simulink model "EKF"  (R2018b)
settings: Solver=ode45  StartTime=0.0  StopTime=900  MaxStep=0.001  RelTol=1e-3
libraries: simulink x9
settings Model: Creator=LaAir  LastModifiedBy=LaAir

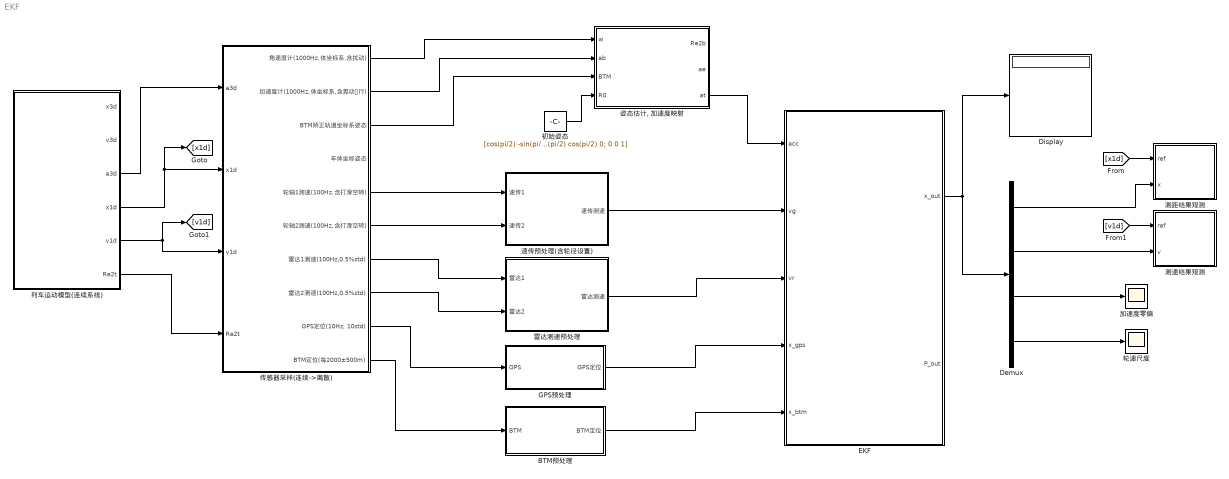
== system EKF ==
  BTM预处理 : Subsystem
  Demux : Demux
  Display : Display
  EKF : MATLAB Function  TreatAsAtomicUnit=on  SystemSampleTime=1e-3
  GPS预处理 : Subsystem
  传感器采样(连续->离散) : Subsystem
  列车运动模型(连续系统) : Subsystem
  初始姿态 : Constant  Value=[cos(pi/2) -sin(pi/2) 0; sin(pi/2) cos(pi/2) 0; 0 0 1]
  加速度零偏 : Scope
  "姿态估计, 加速度映射" : Subsystem
  测距结果观测 : Subsystem
  测速结果观测 : Subsystem
  轮速尺度 : Scope
  速传预处理(含轮径设置) : Subsystem
  雷达测速预处理 : Subsystem
  wires:
  速传预处理(含轮径设置)/1(速传测速) -> EKF/2(vg)
  雷达测速预处理/1(雷达测速) -> EKF/3(vr)
  BTM预处理/1(BTM定位) -> EKF/5(x_btm)
  GPS预处理/1(GPS定位) -> EKF/4(x_gps)
  列车运动模型(连续系统)/5(v1d) -> [v1d], 传感器采样(连续->离散)/3(v1d)
  列车运动模型(连续系统)/4(x1d) -> 传感器采样(连续->离散)/2(x1d), [x1d]
  列车运动模型(连续系统)/3(a3d) -> 传感器采样(连续->离散)/1(a3d)
  传感器采样(连续->离散)/5(轮轴1测速(100Hz,含打滑空转)) -> 速传预处理(含轮径设置)/1(速传1)
  传感器采样(连续->离散)/10(BTM定位(每2000±500m)) -> BTM预处理/1(BTM)
  列车运动模型(连续系统)/6(Re2t) -> 传感器采样(连续->离散)/4(Re2t)
  传感器采样(连续->离散)/9("GPS定位(10Hz, 10std)") -> GPS预处理/1(GPS)
  传感器采样(连续->离散)/7(雷达1测速(100Hz,0.5%std)) -> 雷达测速预处理/1(雷达1)
  传感器采样(连续->离散)/6(轮轴2测速(100Hz,含打滑空转)) -> 速传预处理(含轮径设置)/2(速传2)
  传感器采样(连续->离散)/8(雷达2测速(100Hz,0.5%std)) -> 雷达测速预处理/2(雷达2)
  初始姿态/1 -> "姿态估计, 加速度映射"/4(R0)
  传感器采样(连续->离散)/1(角速度计(1000Hz,体坐标系,含扰动)) -> "姿态估计, 加速度映射"/1(w)
  传感器采样(连续->离散)/2(加速度计(1000Hz,体坐标系,含晃动🐍行)) -> "姿态估计, 加速度映射"/2(ab)
  传感器采样(连续->离散)/3(BTM矫正轨道坐标系姿态) -> "姿态估计, 加速度映射"/3(BTM)
  EKF/1(x_out) -> Demux/1, Display/1
  [x1d] -> 测距结果观测/1(ref)
  [v1d] -> 测速结果观测/1(ref)
  Demux/1 -> 测距结果观测/2(x)
  Demux/2 -> 测速结果观测/2(v)
  Demux/3 -> 加速度零偏/1
  Demux/4 -> 轮速尺度/1
  "姿态估计, 加速度映射"/3(at) -> EKF/1(acc)

== system EKF/BTM预处理 ==
  note: 需将最后输出的采样频率与主融合器保持一致(1000Hz)
  BTM : Inport
  1000Hz : ZeroOrderHold  SampleTime=1e-3
  Pulse Holder (1000Hz) : Subsystem
  BTM定位 : Outport
  wires:
  BTM/1 -> 1000Hz/1
  1000Hz/1 -> Pulse Holder (1000Hz)/1(I)
  Pulse Holder (1000Hz)/1(O) -> BTM定位/1

== system EKF/GPS预处理 ==
  note: 需将最后输出的采样频率与主融合器保持一致(1000Hz)
  GPS : Inport
  Pulse Holder (1000Hz) : Subsystem
  GPS定位 : Outport
  wires:
  GPS/1 -> Pulse Holder (1000Hz)/1(I)
  Pulse Holder (1000Hz)/1(O) -> GPS定位/1

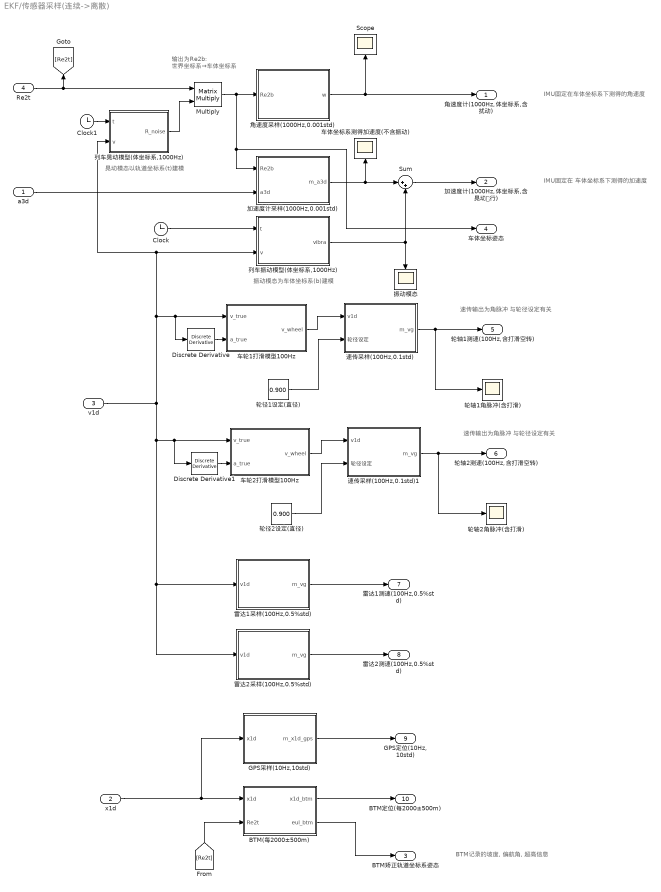
== system EKF/传感器采样(连续->离散) ==
  note: 速传输出为角脉冲
      | 与轮径设定有关
  note: 速传输出为角脉冲
      | 与轮径设定有关
  note: 输出为Re2b:
      | 世界坐标系→车体坐标系
  note: IMU固定在车体坐标系下测得的角速度
  note: IMU固定在 车体坐标系下测得的加速度
  note: 振动模态为车体坐标系(b)建模
  note: 晃动模态以轨道坐标系(t)建模
  note: BTM记录的坡度, 偏航角, 超高信息
  a3d : Inport
  x1d : Inport  Port=2
  v1d : Inport  Port=3
  Re2t : Inport  Port=4
  BTM(每2000±500m) : Subsystem
  Clock : Clock
  Clock1 : Clock
  Discrete Derivative : simulink/Discrete/Discrete Derivative  gainval=1.0  ICPrevScaledInput=0.0  OutMin=[]  OutMax=[]  OutDataType=fixdt(1, 16)  OutScaling=2^-10  DoSatur=off
  Discrete Derivative1 : simulink/Discrete/Discrete Derivative  gainval=1.0  ICPrevScaledInput=0.0  OutMin=[]  OutMax=[]  OutDataType=fixdt(1, 16)  OutScaling=2^-10  DoSatur=off
  GPS采样(10Hz,10std) : Subsystem
  Multiply : Product  Multiplication=Matrix(*)
  Scope : Scope
  Sum : Sum  Inputs=|++
  列车振动模型(体坐标系,1000Hz) : MATLAB Function  TreatAsAtomicUnit=on  SystemSampleTime=1e-3
  列车晃动模型(体坐标系,1000Hz) : MATLAB Function  TreatAsAtomicUnit=on  SystemSampleTime=1e-3
  加速度计采样(1000Hz,0.001std) : Subsystem
  振动模态 : Scope
  角速度采样(1000Hz,0.001std) : Subsystem
  车体坐标系测得加速度(不含振动) : Scope
  车轮1打滑模型100Hz : MATLAB Function  TreatAsAtomicUnit=on  SystemSampleTime=1e-2
  车轮2打滑模型100Hz : MATLAB Function  TreatAsAtomicUnit=on  SystemSampleTime=1e-2
  轮径1设定(直径) : Constant  Value=0.900
  轮径2设定(直径) : Constant  Value=0.900
  轮轴1角脉冲(含打滑) : Scope
  轮轴2角脉冲(含打滑) : Scope
  速传采样(100Hz,0.1std) : Subsystem
  速传采样(100Hz,0.1std)1 : Subsystem
  雷达1采样(100Hz,0.5%std) : Subsystem
  雷达2采样(100Hz,0.5%std) : Subsystem
  角速度计(1000Hz,体坐标系,含扰动) : Outport
  加速度计(1000Hz,体坐标系,含晃动🐍行) : Outport  Port=2
  BTM矫正轨道坐标系姿态 : Outport  Port=3
  车体坐标姿态 : Outport  Port=4
  轮轴1测速(100Hz,含打滑空转) : Outport  Port=5
  轮轴2测速(100Hz,含打滑空转) : Outport  Port=6
  雷达1测速(100Hz,0.5%std) : Outport  Port=7
  雷达2测速(100Hz,0.5%std) : Outport  Port=8
  "GPS定位(10Hz, 10std)" : Outport  Port=9
  BTM定位(每2000±500m) : Outport  Port=10
  wires:
  x1d/1 -> GPS采样(10Hz,10std)/1(x1d), BTM(每2000±500m)/1(x1d)
  BTM(每2000±500m)/1(x1d_btm) -> BTM定位(每2000±500m)/1
  速传采样(100Hz,0.1std)/1(m_vg) -> 轮轴1角脉冲(含打滑)/1, 轮轴1测速(100Hz,含打滑空转)/1
  GPS采样(10Hz,10std)/1(m_x1d_gps) -> "GPS定位(10Hz, 10std)"/1
  a3d/1 -> 加速度计采样(1000Hz,0.001std)/2(a3d)
  轮径1设定(直径)/1 -> 速传采样(100Hz,0.1std)/2(轮径设定)
  雷达1采样(100Hz,0.5%std)/1(m_vg) -> 雷达1测速(100Hz,0.5%std)/1
  Discrete Derivative/1 -> 车轮1打滑模型100Hz/2(a_true)
  车轮1打滑模型100Hz/1(v_wheel) -> 速传采样(100Hz,0.1std)/1(v1d)
  Clock/1 -> 列车振动模型(体坐标系,1000Hz)/1(t)
  加速度计采样(1000Hz,0.001std)/1(m_a3d) -> 车体坐标系测得加速度(不含振动)/1, Sum/1
  Sum/1 -> 加速度计(1000Hz,体坐标系,含晃动🐍行)/1
  列车振动模型(体坐标系,1000Hz)/1(vibra) -> Sum/2, 振动模态/1
  车轮2打滑模型100Hz/1(v_wheel) -> 速传采样(100Hz,0.1std)1/1(v1d)
  轮径2设定(直径)/1 -> 速传采样(100Hz,0.1std)1/2(轮径设定)
  Discrete Derivative1/1 -> 车轮2打滑模型100Hz/2(a_true)
  速传采样(100Hz,0.1std)1/1(m_vg) -> 轮轴2角脉冲(含打滑)/1, 轮轴2测速(100Hz,含打滑空转)/1
  v1d/1 -> Discrete Derivative1/1, 车轮2打滑模型100Hz/1(v_true), 雷达2采样(100Hz,0.5%std)/1(v1d), 雷达1采样(100Hz,0.5%std)/1(v1d), 列车晃动模型(体坐标系,1000Hz)/2(v), 列车振动模型(体坐标系,1000Hz)/2(v), Discrete Derivative/1, 车轮1打滑模型100Hz/1(v_true)
  雷达2采样(100Hz,0.5%std)/1(m_vg) -> 雷达2测速(100Hz,0.5%std)/1
  Re2t/1 -> Multiply/1, [Re2t]
  列车晃动模型(体坐标系,1000Hz)/1(R_noise) -> Multiply/2
  Clock1/1 -> 列车晃动模型(体坐标系,1000Hz)/1(t)
  Multiply/1 -> 角速度采样(1000Hz,0.001std)/1(Re2b), 车体坐标姿态/1, 加速度计采样(1000Hz,0.001std)/1(Re2b)
  角速度采样(1000Hz,0.001std)/1(w) -> 角速度计(1000Hz,体坐标系,含扰动)/1, Scope/1
  BTM(每2000±500m)/2(eul_btm) -> BTM矫正轨道坐标系姿态/1
  [Re2t] -> BTM(每2000±500m)/2(Re2t)

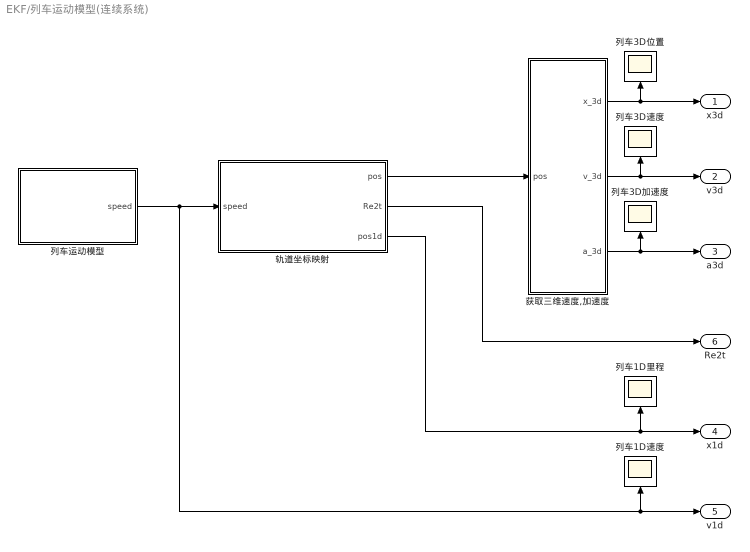
== system EKF/列车运动模型(连续系统) ==
  列车1D速度 : Scope
  列车1D里程 : Scope
  列车3D位置 : Scope
  列车3D加速度 : Scope
  列车3D速度 : Scope
  列车运动模型 : Subsystem
  获取三维速度,加速度 : Subsystem
  轨道坐标映射 : Subsystem
  x3d : Outport
  v3d : Outport  Port=2
  a3d : Outport  Port=3
  x1d : Outport  Port=4
  v1d : Outport  Port=5
  Re2t : Outport  Port=6
  wires:
  轨道坐标映射/1(pos) -> 获取三维速度,加速度/1(pos)
  获取三维速度,加速度/1(x_3d) -> 列车3D位置/1, x3d/1
  列车运动模型/1(speed) -> 轨道坐标映射/1(speed), 列车1D速度/1, v1d/1
  获取三维速度,加速度/3(a_3d) -> 列车3D加速度/1, a3d/1
  获取三维速度,加速度/2(v_3d) -> 列车3D速度/1, v3d/1
  轨道坐标映射/3(pos1d) -> x1d/1, 列车1D里程/1
  轨道坐标映射/2(Re2t) -> Re2t/1

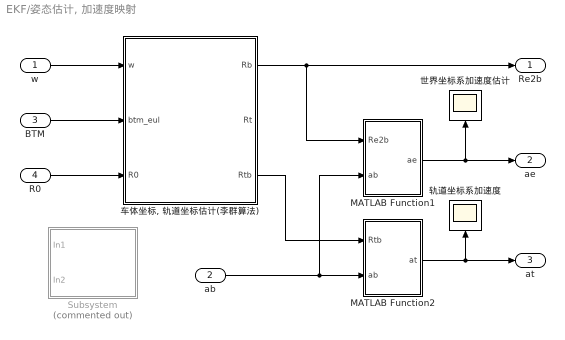
== system EKF/姿态估计, 加速度映射 ==
  w : Inport
  ab : Inport  Port=2
  BTM : Inport  Port=3
  R0 : Inport  Port=4
  MATLAB Function1 : MATLAB Function  TreatAsAtomicUnit=on
  MATLAB Function2 : MATLAB Function  TreatAsAtomicUnit=on
  Subsystem : Subsystem  Commented=on
  世界坐标系加速度估计 : Scope
  "车体坐标, 轨道坐标估计(李群算法)" : MATLAB Function  TreatAsAtomicUnit=on  SystemSampleTime=1e-3
  轨道坐标系加速度 : Scope
  Re2b : Outport
  ae : Outport  Port=2
  at : Outport  Port=3
  wires:
  "车体坐标, 轨道坐标估计(李群算法)"/1(Rb) -> Re2b/1, MATLAB Function1/1(Re2b)
  ab/1 -> MATLAB Function2/2(ab), MATLAB Function1/2(ab)
  R0/1 -> "车体坐标, 轨道坐标估计(李群算法)"/3(R0)
  w/1 -> "车体坐标, 轨道坐标估计(李群算法)"/1(w)
  BTM/1 -> "车体坐标, 轨道坐标估计(李群算法)"/2(btm_eul)
  MATLAB Function1/1(ae) -> ae/1, 世界坐标系加速度估计/1
  "车体坐标, 轨道坐标估计(李群算法)"/3(Rtb) -> MATLAB Function2/1(Rtb)
  MATLAB Function2/1(at) -> at/1, 轨道坐标系加速度/1

== system EKF/测距结果观测 ==
  ref : Inport
  x : Inport  Port=2
  BTM开窗失败 : MATLAB Function  TreatAsAtomicUnit=on
  EKF测距偏差 : Scope
  EKF测距对比 : Scope  NumInputPorts=2
  Scope : Scope
  Sum : Sum  Inputs=+-
  wires:
  x/1 -> EKF测距对比/2, Sum/2
  Sum/1 -> BTM开窗失败/1(u), EKF测距偏差/1
  ref/1 -> Sum/1, EKF测距对比/1
  BTM开窗失败/1(y) -> Scope/1

== system EKF/测速结果观测 ==
  ref : Inport
  v : Inport  Port=2
  EKF测速偏差 : Scope
  EKF速度对比 : Scope  NumInputPorts=2
  Sum : Sum  Inputs=+-
  wires:
  v/1 -> EKF速度对比/2, Sum/2
  Sum/1 -> EKF测速偏差/1
  ref/1 -> Sum/1, EKF速度对比/1

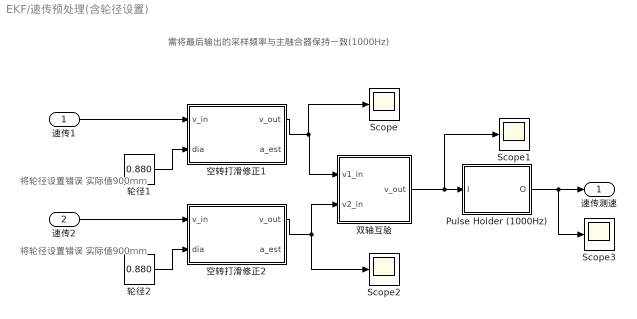
== system EKF/速传预处理(含轮径设置) ==
  note: 将轮径设置错误
      | 实际值900mm
  note: 将轮径设置错误
      | 实际值900mm
  note: 需将最后输出的采样频率与主融合器保持一致(1000Hz)
  速传1 : Inport
  速传2 : Inport  Port=2
  Pulse Holder (1000Hz) : Subsystem
  Scope{,1..3} (4 alike) : Scope
  双轴互验 : MATLAB Function  TreatAsAtomicUnit=on  SystemSampleTime=1e-2
  空转打滑修正1 : MATLAB Function  TreatAsAtomicUnit=on  SystemSampleTime=1e-2
  空转打滑修正2 : MATLAB Function  TreatAsAtomicUnit=on  SystemSampleTime=1e-2
  轮径1 : Constant  Value=0.880
  轮径2 : Constant  Value=0.880
  速传测速 : Outport
  wires:
  轮径1/1 -> 空转打滑修正1/2(dia)
  空转打滑修正2/1(v_out) -> Scope2/1, 双轴互验/2(v2_in)
  双轴互验/1(v_out) -> Scope1/1, Pulse Holder (1000Hz)/1(I)
  空转打滑修正1/1(v_out) -> Scope/1, 双轴互验/1(v1_in)
  轮径2/1 -> 空转打滑修正2/2(dia)
  速传1/1 -> 空转打滑修正1/1(v_in)
  速传2/1 -> 空转打滑修正2/1(v_in)
  Pulse Holder (1000Hz)/1(O) -> Scope3/1, 速传测速/1

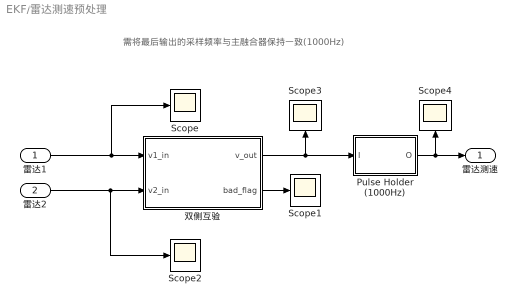
== system EKF/雷达测速预处理 ==
  note: 需将最后输出的采样频率与主融合器保持一致(1000Hz)
  雷达1 : Inport
  雷达2 : Inport  Port=2
  Pulse Holder (1000Hz) : Subsystem
  Scope{,1..4} (5 alike) : Scope
  双侧互验 : MATLAB Function  TreatAsAtomicUnit=on  SystemSampleTime=1e-2
  雷达测速 : Outport
  wires:
  雷达1/1 -> 双侧互验/1(v1_in), Scope/1
  雷达2/1 -> Scope2/1, 双侧互验/2(v2_in)
  双侧互验/1(v_out) -> Scope3/1, Pulse Holder (1000Hz)/1(I)
  双侧互验/2(bad_flag) -> Scope1/1
  Pulse Holder (1000Hz)/1(O) -> 雷达测速/1, Scope4/1

== system EKF/BTM预处理/Pulse Holder (1000Hz) ==
  I : Inport
  Multiply : Product
  pulse holder : Subsystem
  O : Outport
  wires:
  Multiply/1 -> O/1
  pulse holder/1(O) -> Multiply/2
  I/1 -> Multiply/1, pulse holder/1(I)

== system EKF/GPS预处理/Pulse Holder (1000Hz) ==
  I : Inport
  Multiply : Product
  pulse holder : Subsystem
  O : Outport
  wires:
  Multiply/1 -> O/1
  pulse holder/1(O) -> Multiply/2
  I/1 -> Multiply/1, pulse holder/1(I)

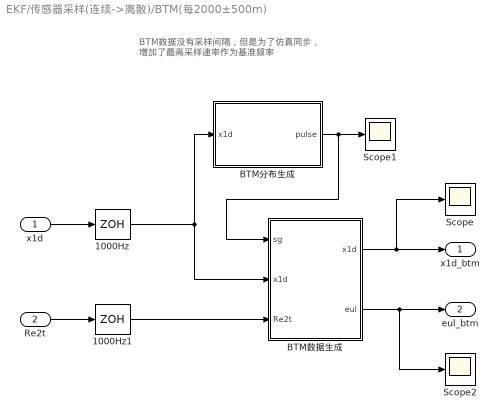
== system EKF/传感器采样(连续->离散)/BTM(每2000±500m) ==
  note: BTM数据没有采样间隔，但是为了仿真同步，
      | 增加了最高采样速率作为基准频率
  x1d : Inport
  Re2t : Inport  Port=2
  1000Hz : ZeroOrderHold  SampleTime=1e-3
  1000Hz1 : ZeroOrderHold  SampleTime=1e-3
  BTM分布生成 : MATLAB Function  TreatAsAtomicUnit=on  SystemSampleTime=1e-3
  BTM数据生成 : MATLAB Function  TreatAsAtomicUnit=on  SystemSampleTime=1e-3
  Scope : Scope
  Scope1 : Scope
  Scope2 : Scope
  x1d_btm : Outport
  eul_btm : Outport  Port=2
  wires:
  x1d/1 -> 1000Hz/1
  1000Hz/1 -> BTM数据生成/2("x1d "), BTM分布生成/1(x1d)
  Re2t/1 -> 1000Hz1/1
  BTM分布生成/1(pulse) -> BTM数据生成/1(sg), Scope1/1
  1000Hz1/1 -> BTM数据生成/3(Re2t)
  BTM数据生成/1(x1d) -> Scope/1, x1d_btm/1
  BTM数据生成/2(eul) -> Scope2/1, eul_btm/1

== system EKF/传感器采样(连续->离散)/GPS采样(10Hz,10std) ==
  x1d : Inport
  "10Hz, 10std" : simulink/Sources/Band-Limited White Noise  Cov=10  Ts=1e-1  seed=1006
  10hz采样 : ZeroOrderHold  SampleTime=1e-1
  GPS定位(10Hz,10std) : Scope
  Sum : Sum
  m_x1d_gps : Outport
  wires:
  x1d/1 -> 10hz采样/1
  "10Hz, 10std"/1 -> Sum/1
  10hz采样/1 -> Sum/2
  Sum/1 -> GPS定位(10Hz,10std)/1, m_x1d_gps/1

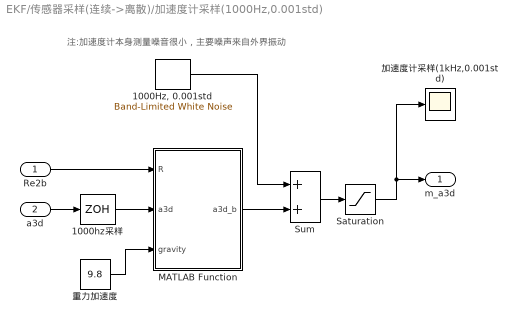
== system EKF/传感器采样(连续->离散)/加速度计采样(1000Hz,0.001std) ==
  note: 注:加速度计本身测量噪音很小，主要噪声来自外界振动
  Re2b : Inport
  a3d : Inport  Port=2
  "1000Hz, 0.001std" : simulink/Sources/Band-Limited White Noise  Cov=1e-9  Ts=1e-3  seed=1001
  1000hz采样 : ZeroOrderHold  SampleTime=1e-3
  MATLAB Function : MATLAB Function  TreatAsAtomicUnit=on
  Saturation : Saturate  UpperLimit=100  LowerLimit=-100
  Sum : Sum
  加速度计采样(1kHz,0.001std) : Scope
  重力加速度 : Constant  Value=9.8
  m_a3d : Outport
  wires:
  "1000Hz, 0.001std"/1 -> Sum/1
  MATLAB Function/1(a3d_b) -> Sum/2
  Sum/1 -> Saturation/1
  Re2b/1 -> MATLAB Function/1(R)
  a3d/1 -> 1000hz采样/1
  1000hz采样/1 -> MATLAB Function/2(a3d)
  重力加速度/1 -> MATLAB Function/3(gravity)
  Saturation/1 -> m_a3d/1, 加速度计采样(1kHz,0.001std)/1

== system EKF/传感器采样(连续->离散)/角速度采样(1000Hz,0.001std) ==
  Re2b : Inport
  "1000Hz, 1e-3std" : simulink/Sources/Band-Limited White Noise  Cov=1e-9  Ts=1e-3  seed=1010
  Sum1 : Sum
  角速度采样(1000Hz) : MATLAB Function  TreatAsAtomicUnit=on  SystemSampleTime=1e-3
  w : Outport
  wires:
  "1000Hz, 1e-3std"/1 -> Sum1/1
  角速度采样(1000Hz)/1(w) -> Sum1/2
  Sum1/1 -> w/1
  Re2b/1 -> 角速度采样(1000Hz)/1(R)

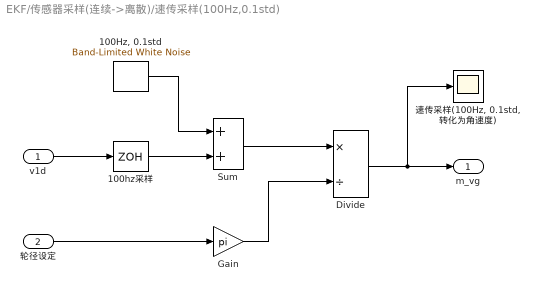
== system EKF/传感器采样(连续->离散)/速传采样(100Hz,0.1std) ==
  v1d : Inport
  轮径设定 : Inport  Port=2
  "100Hz, 0.1std" : simulink/Sources/Band-Limited White Noise  Cov=1e-4  Ts=1e-2  seed=1002
  100hz采样 : ZeroOrderHold  SampleTime=1e-2
  Divide : Product  Inputs=*/
  Gain : Gain  Gain=pi
  Sum : Sum
  "速传采样(100Hz, 0.1std, 转化为角速度)" : Scope
  m_vg : Outport
  wires:
  v1d/1 -> 100hz采样/1
  100hz采样/1 -> Sum/2
  Sum/1 -> Divide/1
  "100Hz, 0.1std"/1 -> Sum/1
  Divide/1 -> "速传采样(100Hz, 0.1std, 转化为角速度)"/1, m_vg/1
  Gain/1 -> Divide/2
  轮径设定/1 -> Gain/1

== system EKF/传感器采样(连续->离散)/速传采样(100Hz,0.1std)1 ==
  v1d : Inport
  轮径设定 : Inport  Port=2
  "100Hz, 0.1std" : simulink/Sources/Band-Limited White Noise  Cov=1e-4  Ts=1e-2  seed=1003
  100hz采样 : ZeroOrderHold  SampleTime=1e-2
  Divide : Product  Inputs=*/
  Gain : Gain  Gain=pi
  Sum : Sum
  "速传采样(100Hz, 0.1std, 转化为角速度)" : Scope
  m_vg : Outport
  wires:
  v1d/1 -> 100hz采样/1
  100hz采样/1 -> Sum/2
  Sum/1 -> Divide/1
  "100Hz, 0.1std"/1 -> Sum/1
  Divide/1 -> "速传采样(100Hz, 0.1std, 转化为角速度)"/1, m_vg/1
  Gain/1 -> Divide/2
  轮径设定/1 -> Gain/1

== system EKF/传感器采样(连续->离散)/雷达1采样(100Hz,0.5%std) ==
  v1d : Inport
  "100Hz, 0.005std" : simulink/Sources/Band-Limited White Noise  Cov=25e-8  Ts=1e-2  seed=1004
  100hz采样 : ZeroOrderHold  SampleTime=1e-2
  Multiply : Product
  Sum : Sum
  "速传采样(100Hz, 0.5%std)" : Scope
  m_vg : Outport
  wires:
  v1d/1 -> 100hz采样/1
  100hz采样/1 -> Multiply/2, Sum/2
  Sum/1 -> "速传采样(100Hz, 0.5%std)"/1, m_vg/1
  "100Hz, 0.005std"/1 -> Multiply/1
  Multiply/1 -> Sum/1

== system EKF/传感器采样(连续->离散)/雷达2采样(100Hz,0.5%std) ==
  v1d : Inport
  "100Hz, 0.005std" : simulink/Sources/Band-Limited White Noise  Cov=25e-8  Ts=1e-2  seed=1005
  100hz采样 : ZeroOrderHold  SampleTime=1e-2
  Multiply : Product
  Sum : Sum
  "速传采样(100Hz, 0.5%std)" : Scope
  m_vg : Outport
  wires:
  v1d/1 -> 100hz采样/1
  100hz采样/1 -> Multiply/2, Sum/2
  Sum/1 -> "速传采样(100Hz, 0.5%std)"/1, m_vg/1
  "100Hz, 0.005std"/1 -> Multiply/1
  Multiply/1 -> Sum/1

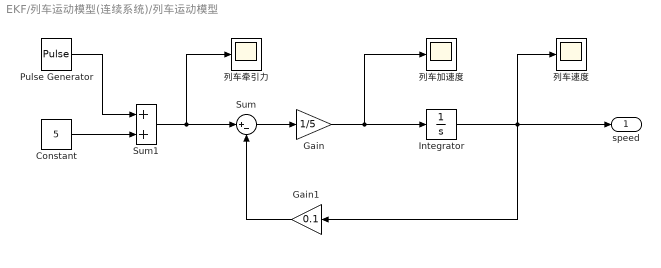
== system EKF/列车运动模型(连续系统)/列车运动模型 ==
  Constant : Constant  Value=5
  Gain : Gain  Gain=1/5
  Gain1 : Gain  Gain=0.1
  Integrator : Integrator
  Pulse Generator : DiscretePulseGenerator  PulseType=Time based  Amplitude=5  Period=600  PulseWidth=50
  Sum : Sum  Inputs=|+-
  Sum1 : Sum
  列车加速度 : Scope
  列车牵引力 : Scope
  列车速度 : Scope
  speed : Outport
  wires:
  Gain1/1 -> Sum/2
  Integrator/1 -> 列车速度/1, speed/1, Gain1/1
  Sum/1 -> Gain/1
  Gain/1 -> 列车加速度/1, Integrator/1
  Pulse Generator/1 -> Sum1/1
  Sum1/1 -> 列车牵引力/1, Sum/1
  Constant/1 -> Sum1/2

== system EKF/列车运动模型(连续系统)/获取三维速度,加速度 ==
  pos : Inport
  Derivative : Derivative
  Derivative1 : Derivative
  x_3d : Outport
  v_3d : Outport  Port=2
  a_3d : Outport  Port=3
  wires:
  Derivative/1 -> v_3d/1, Derivative1/1
  Derivative1/1 -> a_3d/1
  pos/1 -> x_3d/1, Derivative/1

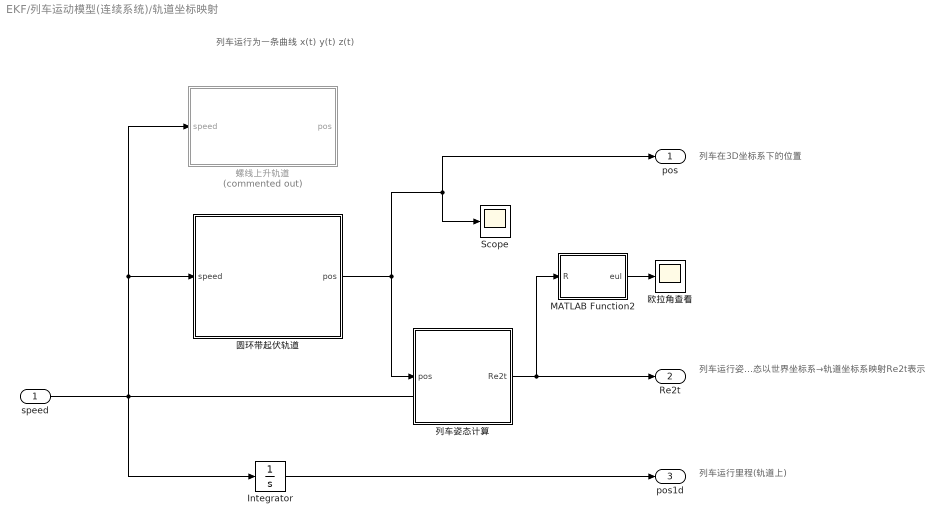
== system EKF/列车运动模型(连续系统)/轨道坐标映射 ==
  note: 列车运行为一条曲线
      | x(t) y(t) z(t)
  note: 列车运行里程(轨道上)
  note: 列车在3D坐标系下的位置
  note: 列车运行姿态以世界坐标系→轨道坐标系映射Re2t表示
  speed : Inport
  Integrator : Integrator
  MATLAB Function2 : MATLAB Function  TreatAsAtomicUnit=on
  Scope : Scope
  列车姿态计算 : Subsystem
  圆环带起伏轨道 : Subsystem
  欧拉角查看 : Scope
  螺线上升轨道 : Subsystem  Commented=on
  pos : Outport
  Re2t : Outport  Port=2
  pos1d : Outport  Port=3
  wires:
  speed/1 -> 螺线上升轨道/1(speed), 圆环带起伏轨道/1(speed), Integrator/1
  圆环带起伏轨道/1(pos) -> 列车姿态计算/1(pos), Scope/1, pos/1
  Integrator/1 -> pos1d/1
  列车姿态计算/1(Re2t) -> Re2t/1, MATLAB Function2/1(R)
  MATLAB Function2/1(eul) -> 欧拉角查看/1

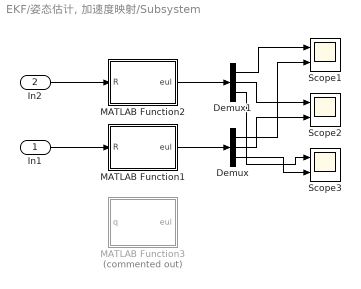
== system EKF/姿态估计, 加速度映射/Subsystem ==
  In1 : Inport
  In2 : Inport  Port=2
  Demux : Demux  Outputs=3
  Demux1 : Demux  Outputs=3
  MATLAB Function1 : MATLAB Function  TreatAsAtomicUnit=on
  MATLAB Function2 : MATLAB Function  TreatAsAtomicUnit=on
  MATLAB Function3 : MATLAB Function  Commented=on  TreatAsAtomicUnit=on
  Scope1 : Scope  NumInputPorts=2
  Scope2 : Scope  NumInputPorts=2
  Scope3 : Scope  NumInputPorts=2
  wires:
  Demux/1 -> Scope1/2
  Demux/3 -> Scope3/2
  MATLAB Function1/1(eul) -> Demux/1
  In2/1 -> MATLAB Function2/1(R)
  MATLAB Function2/1(eul) -> Demux1/1
  Demux1/1 -> Scope1/1
  Demux1/3 -> Scope3/1
  Demux1/2 -> Scope2/1
  Demux/2 -> Scope2/2
  In1/1 -> MATLAB Function1/1(R)

== system EKF/速传预处理(含轮径设置)/Pulse Holder (1000Hz) ==
  I : Inport
  Multiply : Product
  pulse holder : Subsystem
  O : Outport
  wires:
  Multiply/1 -> O/1
  pulse holder/1(O) -> Multiply/2
  I/1 -> Multiply/1, pulse holder/1(I)

== system EKF/雷达测速预处理/Pulse Holder (1000Hz) ==
  I : Inport
  Multiply : Product
  pulse holder : Subsystem
  O : Outport
  wires:
  Multiply/1 -> O/1
  pulse holder/1(O) -> Multiply/2
  I/1 -> Multiply/1, pulse holder/1(I)

== system EKF/BTM预处理/Pulse Holder (1000Hz)/pulse holder ==
  I : Inport
  1000Hz : ZeroOrderHold  SampleTime=1e-3
  MATLAB Function : MATLAB Function  TreatAsAtomicUnit=on
  Sum : Sum  Inputs=+-
  Unit Delay : UnitDelay  SampleTime=-1
  O : Outport
  wires:
  MATLAB Function/1(y) -> O/1
  Sum/1 -> MATLAB Function/1(u)
  1000Hz/1 -> Unit Delay/1, Sum/1
  I/1 -> 1000Hz/1
  Unit Delay/1 -> Sum/2

== system EKF/GPS预处理/Pulse Holder (1000Hz)/pulse holder ==
  I : Inport
  1000Hz : ZeroOrderHold  SampleTime=1e-3
  MATLAB Function : MATLAB Function  TreatAsAtomicUnit=on
  Sum : Sum  Inputs=+-
  Unit Delay : UnitDelay  SampleTime=-1
  O : Outport
  wires:
  MATLAB Function/1(y) -> O/1
  Sum/1 -> MATLAB Function/1(u)
  1000Hz/1 -> Unit Delay/1, Sum/1
  I/1 -> 1000Hz/1
  Unit Delay/1 -> Sum/2

== system EKF/列车运动模型(连续系统)/轨道坐标映射/列车姿态计算 ==
  pos : Inport
  Derivative : Derivative  CoefficientInTFapproximation=100
  Derivative1 : Derivative  CoefficientInTFapproximation=100
  MATLAB Function : MATLAB Function  TreatAsAtomicUnit=on
  MATLAB Function3 : MATLAB Function  TreatAsAtomicUnit=on
  Transfer Fcn : TransferFcn  Numerator=[10]  Denominator=[1 10]
  Re2t : Outport
  wires:
  MATLAB Function/1(R) -> Re2t/1
  Derivative1/1 -> MATLAB Function3/2(d2)
  pos/1 -> Derivative/1
  Derivative/1 -> MATLAB Function/1(vtan), MATLAB Function3/1(d1), Derivative1/1
  MATLAB Function3/1(roll) -> Transfer Fcn/1
  Transfer Fcn/1 -> MATLAB Function/2(roll)

== system EKF/列车运动模型(连续系统)/轨道坐标映射/圆环带起伏轨道 ==
  note: z(s)=Asin(Lz​2π​s+φ)
      | g(s)=dsdz​=A(Lz​2π​)cos(Lz​2π​s+φ)
  speed : Inport
  Integrator1 : Integrator
  Integrator2 : Integrator
  MATLAB Function1 : MATLAB Function  TreatAsAtomicUnit=on
  pos : Outport
  wires:
  speed/1 -> MATLAB Function1/2(v), Integrator2/1
  Integrator1/1 -> MATLAB Function1/3(theta)
  Integrator2/1 -> MATLAB Function1/1(s)
  MATLAB Function1/1(theta_dot) -> Integrator1/1
  MATLAB Function1/2(pos) -> pos/1

== system EKF/列车运动模型(连续系统)/轨道坐标映射/螺线上升轨道 ==
  speed : Inport
  Integrator : Integrator
  MATLAB Function : MATLAB Function  TreatAsAtomicUnit=on
  pos : Outport
  wires:
  MATLAB Function/1(pos) -> pos/1
  Integrator/1 -> MATLAB Function/1(s)
  speed/1 -> Integrator/1

== system EKF/速传预处理(含轮径设置)/Pulse Holder (1000Hz)/pulse holder ==
  I : Inport
  1000Hz : ZeroOrderHold  SampleTime=1e-3
  MATLAB Function : MATLAB Function  TreatAsAtomicUnit=on
  Sum : Sum  Inputs=+-
  Unit Delay : UnitDelay  SampleTime=-1
  O : Outport
  wires:
  MATLAB Function/1(y) -> O/1
  Sum/1 -> MATLAB Function/1(u)
  1000Hz/1 -> Unit Delay/1, Sum/1
  I/1 -> 1000Hz/1
  Unit Delay/1 -> Sum/2

== system EKF/雷达测速预处理/Pulse Holder (1000Hz)/pulse holder ==
  I : Inport
  1000Hz : ZeroOrderHold  SampleTime=1e-3
  MATLAB Function : MATLAB Function  TreatAsAtomicUnit=on
  Sum : Sum  Inputs=+-
  Unit Delay : UnitDelay  SampleTime=-1
  O : Outport
  wires:
  MATLAB Function/1(y) -> O/1
  Sum/1 -> MATLAB Function/1(u)
  1000Hz/1 -> Unit Delay/1, Sum/1
  I/1 -> 1000Hz/1
  Unit Delay/1 -> Sum/2

== matlab function EKF/传感器采样(连续->离散)/列车晃动模型(体坐标系,1000Hz) ==
  data: t input; R_noise output; v input
function R_noise = fcn(t, v)
% t: 时间(s)   v: 速度(m/s)
% 输出: R_noise (局部->局部有扰动)

    % ----- 相位状态（保证连续） -----
    persistent phi_r phi_p phi_y last_t
    if isempty(last_t)
        phi_r = 0; phi_p = 0; phi_y = 0; last_t = t;
    end
    dt = max(t - last_t, 1e-6);   % 防止0步长
    last_t = t;

    % ----- 速度相关的“幅值 & 频率”模型（可按实测调整/限幅） -----
    % roll（横摇）：频率近似固定，幅值随速增大
    A_roll = deg2rad(0.5 + 0.005*v);                    % rad
    A_roll = min(A_roll, deg2rad(3));                   % 合理上限
    f_roll = 0.8;                                       % Hz

    % pitch（俯仰）：频率近似固定，幅值随速增大
    A_pitch = deg2rad(0.3 + 0.003*v);
    A_pitch = min(A_pitch, deg2rad(1.5));
    f_pitch = 1.5;                                      % Hz

    % yaw（蛇行）：频率随速增加，幅值随速增加
    Lc = 10;                                            % m，特征蛇行波长
    f_yaw = v / (2*pi*Lc);                              % Hz ≈ v/(2πLc)
    f_yaw = min(max(f_yaw, 0.3), 6.0);                  % 合理范围
    A_yaw = deg2rad(0.2 + 0.004*v);
    A_yaw = min(A_yaw, deg2rad(2));

    % ----- 积分频率得到相位（保证连续） -----
    phi_r = wrapPi(phi_r + 2*pi*f_roll*dt);
    phi_p = wrapPi(phi_p + 2*pi*f_pitch*dt);
    phi_y = wrapPi(phi_y + 2*pi*f_yaw*dt);

    % ----- 角度扰动（小角度，单位 rad） -----
    droll  = A_roll  * sin(phi_r);
    dpitch = A_pitch * sin(phi_p);
    dyaw   = A_yaw   * sin(phi_y);

    % ----- ZYX 欧拉 -> 旋转矩阵 -----
    cz = cos(dyaw);  sz = sin(dyaw);
    cy = cos(dpitch); sy = sin(dpitch);
    cx = cos(droll);  sx = sin(droll);

    Rz = [cz -sz 0; sz cz 0; 0 0 1];
    Ry = [cy 0 sy; 0 1 0; -sy 0 cy];
    Rx = [1 0 0; 0 cx -sx; 0 sx cx];

    R_noise = Rz * Ry * Rx;
end

function a = wrapPi(a)
% 把角度包到 [-pi, pi]
    a = mod(a + pi, 2*pi) - pi;
end

== matlab function EKF/传感器采样(连续->离散)/加速度计采样(1000Hz,0.001std)/MATLAB Function ==
  data: R input; a3d_b output; a3d input; gravity input
function a3d_b = fcn(R, a3d, gravity)
a3d(3) = a3d(3)-gravity;
y = R'*a3d;
a3d_b = y;

== matlab function EKF/传感器采样(连续->离散)/BTM(每2000±500m)/BTM数据生成 ==
  data: sg input; x1d input; x1d output; Re2t input; eul output
function [x1d, eul] = fcn(sg, x1d, Re2t)
if (sg > 0.5)
    x1d = x1d;
    [U, ~, V] = svd(Re2t);
    R = U * V';
    yaw = atan2(R(2,1),R(1,1));
    pitch = asin(-R(3,1));
    roll = atan2(R(3,2),R(3,3));
    eul = [yaw, pitch, roll];
else
    x1d = 0;
    eul = [0,0,0];
end
end

== matlab function EKF/传感器采样(连续->离散)/角速度采样(1000Hz,0.001std)/角速度采样(1000Hz) ==
  data: R input; w output
function w = fcn(R)
dt = 1e-3;
persistent R_pre;
if isempty(R_pre)
    R_pre = R;
end

dR = (R - R_pre) / dt;
R_pre = R;
Omega = R' * dR;
w = [Omega(3,2); Omega(1,3); Omega(2,1)];

== matlab function EKF/传感器采样(连续->离散)/列车振动模型(体坐标系,1000Hz) ==
  data: t input; vibra output; v input
function vibra = vibration(t, v)
% 三维振动干扰 (速度依赖)
% 输入:
%   t - 仿真时间 (s)
%   v - 列车速度 (m/s)
% 输出:
%   ax, ay, az - 三个方向的加速度干扰 (m/s^2)

g = 9.81;  % 重力加速度

% ========== X 方向 (纵向) ==========
% 低频 (纵向起伏)
f_x_low = 0.5 + 0.002*v;
amp_x_low = (0.02 + 0.0002*v) * g;
x_low = amp_x_low * sin(2*pi*f_x_low*t);

% 高频 (轮轨冲击)
D = 0.92;   % 轮径 (m)
f_x_high = v / (pi*D);  % 轮对激励频率
amp_x_high = 0.01 * g;
x_high = amp_x_high * sin(2*pi*f_x_high*t);

ax = x_low + x_high;

% ========== Y 方向 (横向) ==========
% 蛇行运动 (速度依赖)
f_y_hunt = 0.3 + 0.004*v;
amp_y_hunt = (0.05 + 0.0005*v) * g;
y_hunt = amp_y_hunt * sin(2*pi*f_y_hunt*t);

% 中频横向不平顺
f_y_mid = v / 80;   % 对应轨道波长 ~80m
amp_y_mid = 0.02 * g;
y_mid = amp_y_mid * sin(2*pi*f_y_mid*t);

ay = y_hunt + y_mid;

% ========== Z 方向 (垂向) ==========
% 中频垂向振动
f_z_mid = v / 40;   % 对应轨道波长 ~40m
amp_z_mid = (0.05 + 0.0003*v) * g;
z_mid = amp_z_mid * sin(2*pi*f_z_mid*t);

% 瞬态冲击 (道岔/隧道)
pulse_interval = 100;  % 每x秒一次
pulse_width    = 0.3; % 持续0.3秒
if mod(t, pulse_interval) < pulse_width
    z_pulse = 0.1 * g + 0.0005*v;
else
    z_pulse = 0;
end

az = z_mid + z_pulse;
% az = z_mid;
vibra = [ax; ay; az];
end

== matlab function EKF/EKF ==
  data: acc input; x_out output; vg input; vr input; x_gps input; x_btm input; P_out output
function [x_out, P_out] = fcn(acc, vg, vr, x_gps, x_btm)
% 状态: x=[ x; v; b_a; s_w ], 位置/速度/加速度零偏/轮速尺度(≈1+ε)
% 缺测用 NaN；兼容旧工程，位置=0/速度=0 也可视为缺测，但做了低速保护避免误杀真零速

dt = 1e-3;

persistent x P inited
if isempty(inited)
    x = [0; 0; 0; 1.0];
    P = diag([100, 10, 0.1, 1e-2]);
    inited = true;
end

% ---------- 观测缺测兼容层 ----------
% 优先 isnan；保留兼容
if nargin < 5, x_btm = NaN; end
if nargin < 4, x_gps = NaN; end

if ~isnan(x_gps) && x_gps==0, x_gps = NaN; end
if ~isnan(x_btm) && x_btm==0, x_btm = NaN; end

% 速度类：0 既可能是真零速也可能是缺测；若当前状态 |v| 明显非零，则把 0 当缺测
v_now = x(2);
if ~isnan(vg) && vg==0 && abs(v_now)>0.2, vg = NaN; end
if ~isnan(vr) && vr==0 && abs(v_now)>0.2, vr = NaN; end

% 加速度预处理
acc_t = acc(1);
if any(isnan(acc_t)), acc_t = 0; end
a = acc_t;   % 已在外部完成姿态投影到轨道切向

% ---------- 过程模型 ----------
% x = [x; v; b_a; s_w]
F = eye(4);
F(1,2) = dt;     % dx/dv
F(2,3) = -dt;    % dv/db_a

% 过程噪声（经验值，可再调）
sigma_a  = 0.6;          % m/s^2  加计噪声等效
sigma_b  = 1e-3;         % (m/s^2)/sqrt(s)  加计零偏随机游走
sigma_sw = 1e-5;         % 轮径尺度随机游走 /sqrt(s)
G = [0.5*dt^2; dt; 0; 0];  % 加速度噪声驱动到 [x;v]
Q = zeros(4);
Q = Q + (sigma_a^2)*(G*G.');
Q(3,3) = Q(3,3) + (sigma_b^2)*dt;
Q(4,4) = Q(4,4) + (sigma_sw^2)*dt;

% 预测
x = [ x(1) + x(2)*dt;
      x(2) + (a - x(3))*dt;
      x(3);
      x(4) ];
P = F*P*F' + Q;

% 保证 s_w 正且不过分跑飞（简单夹紧）
x(4) = max(0.7, min(1.3, x(4)));

% ---------- 观测与更新 ----------
% h(x):
%   GPS:   x
%   BTM:   x
%   轮速:  s_w * v
%   雷达:  v
H_full = [ 1 0 0 0;          % GPS
           1 0 0 0;          % BTM
           0 x(4) 0 x(2);    % 轮速的正确雅可比！！
           0 1   0 0  ];     % 雷达

z_full = [x_gps; x_btm; vg; vr];

% 测量噪声
sigma_gps = 2.0;    % m
sigma_btm = 0.5;    % m
sigma_vr  = 0.25;   % m/s
% 轮速噪声：基线 + 随速度变化；低速时观测对 s_w 不可观/容易滑差，抬高噪声或跳过
v_abs = abs(x(2));
sigma_vg = 0.05 + 5e-3*v_abs;  % m/s
R_full = diag([sigma_gps^2, sigma_btm^2, sigma_vg^2, sigma_vr^2]);

% 低速保护与防滑（关键）：
% 1) |v| 很小 → 不更新轮速项（对 s_w 几乎不可观）
% 2) 残差过大 → 判定打滑，仅临时放大轮速 R，而不是整条观测抛弃
mask = ~isnan(z_full);
if v_abs < 0.2           % 低速阈值，可调
    mask(3) = false;     % 暂不使用轮速
end

if any(mask)
    H = H_full(mask, :);
    z = z_full(mask);
    R = R_full(mask, mask);

    % 非线性观测值
    h = zeros(nnz(mask),1);
    idx = find(mask);
    for k = 1:numel(idx)
        switch idx(k)
            case 1, h(k) = x(1);           % GPS
            case 2, h(k) = x(1);           % BTM
            case 3, h(k) = x(4)*x(2);      % 轮速
            case 4, h(k) = x(2);           % 雷达
        end
    end

    % 残差预计算
    r = z - h;

    % 若包含轮速项，做一次“打滑检测”：|r_vg| > 3σ → 放大该项 R（例如 ×25）
    if any(idx==3)
        pos = find(idx==3,1,'first');           % 轮速在子观测向量的位置
        if abs(r(pos)) > 3*sqrt(R(pos,pos))
            R(pos,pos) = 25*R(pos,pos);         % 软抑制轮速而非丢弃
        end
    end

    % 标准 EKF 更新
    S = H*P*H' + R;
    K = P*H'/S;
    x = x + K*(z - h);
    P = (eye(4) - K*H)*P*(eye(4) - K*H)' + K*R*K';
end

x_out = x;
P_out = P;
end

== matlab function EKF/传感器采样(连续->离散)/车轮1打滑模型100Hz ==
  data: v_true input; v_wheel output; a_true input
function v_wheel = fcn(v_true, a_true)
% v_true : 真实速度
% a_true : 真实加速度 (m/s^2)
% slip_max : 最大滑移率 (e.g. 0.05)
slip_max = 0.05;
% prob : 在加速/制动时发生打滑的概率 (0~1),需要除以采样间隔代表每秒触发率
prob = 0.05/100;  % 100Hz

persistent isSlip slip_sign slip_val
persistent init
if isempty(init)
    rng('shuffle');
    init = true;
end

if isempty(isSlip)
    isSlip = false;
    slip_sign = 0;
    slip_val = 0;
end

% 判断是否触发新一次打滑/空转
if ~isSlip && rand < prob * abs(a_true)
    % 开始一次事件
    isSlip = true;
    slip_sign = sign(a_true);      % +1=空转, -1=打滑
    slip_val = slip_max * rand;    % 随机强度
end

% 模拟持续若干秒（可加一个持续时间计数器）
if isSlip
    v_wheel = v_true * (1 + slip_sign*slip_val);
    % 简单起见，这里在速度下降/上升时结束事件
    if rand < 0.01
        isSlip = false;
    end
else
    v_wheel = v_true;
end

== matlab function EKF/速传预处理(含轮径设置)/空转打滑修正1 ==
  data: v_in input; v_out output; dia input; a_est output
function [v_out, a_est] = fcn(v_in, dia)
% v_in : 当前轮速输入 (m/s)
% dia  : 轮径 (m)

dt = 1e-2;           % 采样周期 0.01 s
window = 0.25;        % 检测窗口长度 (s)
N = round(window/dt); % 窗口内样本数 (0.1/0.01=10)

% 转换成周向速度
v_in = v_in * dia * pi;

persistent v_buf v_prev
if isempty(v_buf)
    v_buf = v_in * ones(1, N);  % 初始化为N个相同值
    v_prev = v_in;
end

% 更新缓冲区（FIFO）
v_buf = [v_buf(2:end), v_in];

% 计算0.1s内平均加速度
a_est = (v_in - v_buf(1)) / (N*dt);

% 阈值判断
if abs(a_est) > 4
    % 异常 -> 融合估计（平滑过渡）
    v_out = v_prev*0.98 + 0.02*v_in;
else
    % 正常 -> 更新
    v_out = v_in;
end

% 更新状态
v_prev = v_out;;

== matlab function EKF/速传预处理(含轮径设置)/双轴互验 ==
  data: v1_in input; v_out output; v2_in input
function v_out = fcn(v1_in, v2_in)
% v1_in, v2_in : 两个轮速传感器输入 (m/s)
% dt           : 采样周期 (s)

dt = 1e-2;             % 采样周期 0.01 s
window = 0.25;          % 检测窗口长度 (s)
N = round(window/dt);  % 窗口长度对应的采样点数
Th = 3;                % 加速度阈值 (m/s^2)

% 状态变量
persistent v1_buf v2_buf v_prev
if isempty(v1_buf)
    v1_buf = v1_in * ones(1, N);
    v2_buf = v2_in * ones(1, N);
    v_prev = (v1_in + v2_in)/2;
end

% 更新缓冲区（FIFO）
v1_buf = [v1_buf(2:end), v1_in];
v2_buf = [v2_buf(2:end), v2_in];

% 计算0.1s平均加速度
a1 = (v1_in - v1_buf(1)) / (N*dt);
a2 = (v2_in - v2_buf(1)) / (N*dt);

% 判断是否异常
bad1 = abs(a1) > Th;
bad2 = abs(a2) > Th;

% 融合逻辑
if ~bad1 && ~bad2
    v_raw = 0.5*(v1_in + v2_in);   % 两个都正常 → 平均
elseif ~bad1 && bad2
    v_raw = v1_in;                 % 只轮1正常
elseif bad1 && ~bad2
    v_raw = v2_in;                 % 只轮2正常
else
    % 两个都坏 → 融合后平滑过渡
    v_raw = v_prev*0.98 + 0.02*0.5*(v1_in + v2_in);
end

% 输出并更新
v_out  = v_raw;
v_prev = v_out;

== matlab function EKF/速传预处理(含轮径设置)/空转打滑修正2 ==
  data: v_in input; v_out output; dia input; a_est output
function [v_out, a_est] = fcn(v_in, dia)
% v_in : 当前轮速输入 (m/s)
% dia  : 轮径 (m)

dt = 1e-2;           % 采样周期 0.01 s
window = 0.25;        % 检测窗口长度 (s)
N = round(window/dt); % 窗口内样本数 (0.1/0.01=10)

% 转换成周向速度
v_in = v_in * dia * pi;

persistent v_buf v_prev
if isempty(v_buf)
    v_buf = v_in * ones(1, N);  % 初始化为N个相同值
    v_prev = v_in;
end

% 更新缓冲区（FIFO）
v_buf = [v_buf(2:end), v_in];

% 计算0.1s内平均加速度
a_est = (v_in - v_buf(1)) / (N*dt);

% 阈值判断
if abs(a_est) > 4
    % 异常 -> 融合估计（平滑过渡）
    v_out = v_prev*0.98 + 0.02*v_in;
else
    % 正常 -> 更新
    v_out = v_in;
end

% 更新状态
v_prev = v_out;

== matlab function EKF/雷达测速预处理/双侧互验 ==
  data: v1_in input; v_out output; v2_in input; bad_flag output
function [v_out, bad_flag] = fcn(v1_in, v2_in)
if abs(v1_in - v2_in) > 5
    bad_flag = 1;
    v_out = 0;
else
    bad_flag = 0;
    v_out = 0.5*(v1_in + v2_in);
end

end

== matlab function EKF/速传预处理(含轮径设置)/Pulse Holder (1000Hz)/pulse holder/MATLAB Function ==
  data: u input; y output
function y = fcn(u)
if (u ~= 0)
    y=1;
else
    y=0;
end

== matlab function EKF/雷达测速预处理/Pulse Holder (1000Hz)/pulse holder/MATLAB Function ==
  data: u input; y output
function y = fcn(u)
if (u ~= 0)
    y=1;
else
    y=0;
end

== matlab function EKF/BTM预处理/Pulse Holder (1000Hz)/pulse holder/MATLAB Function ==
  data: u input; y output
function y = fcn(u)
if (u ~= 0)
    y=1;
else
    y=0;
end

== matlab function EKF/GPS预处理/Pulse Holder (1000Hz)/pulse holder/MATLAB Function ==
  data: u input; y output
function y = fcn(u)
if (u ~= 0)
    y=1;
else
    y=0;
end

== matlab function EKF/传感器采样(连续->离散)/车轮2打滑模型100Hz ==
  data: v_true input; v_wheel output; a_true input
function v_wheel = fcn(v_true, a_true)
% v_true : 真实速度
% a_true : 真实加速度 (m/s^2)
% slip_max : 最大滑移率 (e.g. 0.05)
slip_max = 0.05;
% prob : 在加速/制动时发生打滑的概率 (0~1),需要除以采样间隔代表每秒触发率
prob = 0.05/100;  % 100Hz

persistent isSlip slip_sign slip_val
persistent init
if isempty(init)
    rng('shuffle');
    init = true;
end

if isempty(isSlip)
    isSlip = false;
    slip_sign = 0;
    slip_val = 0;
end

% 判断是否触发新一次打滑/空转
if ~isSlip && rand < prob * abs(a_true)
    % 开始一次事件
    isSlip = true;
    slip_sign = sign(a_true);      % +1=空转, -1=打滑
    slip_val = slip_max * rand;    % 随机强度
end

% 模拟持续若干秒（可加一个持续时间计数器）
if isSlip
    v_wheel = v_true * (1 + slip_sign*slip_val);
    % 简单起见，这里在速度下降/上升时结束事件
    if rand < 0.01
        isSlip = false;
    end
else
    v_wheel = v_true;
end

== matlab function EKF/列车运动模型(连续系统)/轨道坐标映射/MATLAB Function2 ==
  data: R input; eul output
 function eul = deg(R)
[U, ~, V] = svd(R);
R = U * V';
yaw = atan2(R(2,1),R(1,1));
pitch = asin(-R(3,1));
roll = atan2(R(3,2),R(3,3));
eul = [yaw; pitch; roll]*180/pi;

== matlab function EKF/列车运动模型(连续系统)/轨道坐标映射/列车姿态计算/MATLAB Function ==
  data: vtan input; R output; roll input
function R = fcn(vtan, roll)
% --- 轨道姿态 ---
x_axis = vtan / norm(vtan);            % 切向量 = 局部 x 轴
z_world = [0;0;1];           % 世界竖直方向

% Gram–Schmidt 正交化，得到局部 z 轴 
z_axis = z_world - dot(z_world, x_axis)*x_axis;
z_axis = z_axis / norm(z_axis);

% y 轴由右手定则确定
y_axis = cross(z_axis, x_axis);
y_axis = y_axis / norm(y_axis);

% 以切向量 x_axis 为旋转轴，绕 roll 旋转
K = [ 0  0  0;
      0  0 -1;
      0  1  0 ];
R_roll = eye(3) + sin(roll)*K + (1-cos(roll))*(K*K);

% 世界->轨道 旋转矩阵 (列向量为局部基)
R = [x_axis(:), y_axis(:), z_axis(:)] * R_roll;

== matlab function EKF/列车运动模型(连续系统)/轨道坐标映射/列车姿态计算/MATLAB Function3 ==
  data: d1 input; roll output; d2 input
function roll = fcn(d1, d2)
ds_speed = 75; % 设计速度 75约等于270km/h
r = norm(d1(1:2))^3/norm(d1(1)*d2(2)-d1(2)*d2(1));
g = 9.8;
a = ds_speed^2/r;
a = min(4, a);
roll = atan(a/g);

== matlab function EKF/列车运动模型(连续系统)/轨道坐标映射/圆环带起伏轨道/MATLAB Function1 ==
  data: theta_dot output; s input; pos output; v input; theta input
function [theta_dot, pos] = circleUndulate(s, v, theta)
% s    : 弧长（外部由 v 积分得到）
% v    : 速度
% R    : 半径
R = 10000;
% A,Lz,phi: 起伏参数；Lz列车行进多少米完成一次起伏
A = 20; Lz = 5000; phi = 0;
% theta: 当前角
% z0   : 初始高程基准
z0 = 0;
% 输出:
%   theta_dot = dθ/dt (供外部 Integrator)
%   z_dot     = dz/dt (供外部 Integrator, 可选)
%   x,y,z     = 当前位置

omega = 2*pi / Lz;
z_rel = A * sin(omega*s + phi);                % 相对起伏
g = A * omega * cos(omega*s + phi);            % dz/ds
if abs(g) >= 1
    g = 0.999999 * sign(g);
end

omega_s = sqrt(1 - g*g) / R;                   % dθ/ds
theta_dot = omega_s * v;                       % dθ/dt
% z_dot     = g * v;                             % dz/dt (如果想对 z 再积分)
x = R * cos(theta);
y = R * sin(theta);
z = z0 + z_rel;
pos = [x;y;z];
end

== matlab function EKF/列车运动模型(连续系统)/轨道坐标映射/螺线上升轨道/MATLAB Function ==
  data: s input; pos output
function pos = mapHelix_byGrade(s)
% s     : 沿轨道弧长（由积分器得到）
% R     : 半径 (m)
R = 10000;
% g     : 坡度 = dz/ds（如 2% 取 0.02）
g = 0.02;
% theta0: 初始角 (rad)
theta0 = 0;
% z0    : 初始高度 (m)
z0 = 0;

% 数值保护，避免 |g|>=1
if abs(g) >= 1
    if g >= 0
        g = 1 - 1e-9;
    else
        g = -1 + 1e-9;
    end
end

omega = sqrt(1 - g*g) / R;      % dθ/ds
theta = theta0 + omega .* s;

x = R .* cos(theta);
y = R .* sin(theta);
z = z0 + g .* s;
pos = [x,y,z];
end

== matlab function EKF/测距结果观测/BTM开窗失败 ==
  data: u input; y output
function y = fcn(u)
if abs(u) > 25
    y = 1;
else
    y = 0;
end

== matlab function EKF/姿态估计, 加速度映射/Subsystem/MATLAB Function1 ==
  data: R input; eul output
 function eul = rad(R)
[U, ~, V] = svd(R);
R = U * V';
yaw = atan2(R(2,1),R(1,1));
pitch = asin(-R(3,1));
roll = atan2(R(3,2),R(3,3));
eul = [yaw, pitch, roll];

== matlab function EKF/姿态估计, 加速度映射/MATLAB Function1 ==
  data: Re2b input; ae output; ab input
function ae = fcn(Re2b, ab)
g = 9.8;
ae = Re2b*ab;
ae(3) = ae(3)+g;

== matlab function EKF/姿态估计, 加速度映射/Subsystem/MATLAB Function2 ==
  data: R input; eul output
 function eul = rad(R)
[U, ~, V] = svd(R);
R = U * V';
yaw = atan2(R(2,1),R(1,1));
pitch = asin(-R(3,1));
roll = atan2(R(3,2),R(3,3));
eul = [yaw, pitch, roll];

== matlab function EKF/传感器采样(连续->离散)/BTM(每2000±500m)/BTM分布生成 ==
  data: x1d input; pulse output
function pulse = fcn(x1d)
persistent milestone
if isempty(milestone)
    milestone = 25;
end
if (x1d > milestone)
    pulse = 1;
    milestone = ceil(x1d) + 1500 + randi(1000);
else
    pulse = 0;
end

== matlab function EKF/姿态估计, 加速度映射/Subsystem/MATLAB Function3 ==
  data: q input; eul output
function eul = q2eul(q)
% 输入 q = [qw qx qy qz]，Hamilton 定义（qw 是实部）
% 输出 yaw(Z)、pitch(Y)、roll(X)，单位 rad

    % 拆分
    qw = q(1); qx = q(2); qy = q(3); qz = q(4);

    % 旋转矩阵
    R = [ 1 - 2*(qy^2 + qz^2),   2*(qx*qy - qz*qw),   2*(qx*qz + qy*qw);
          2*(qx*qy + qz*qw),     1 - 2*(qx^2 + qz^2), 2*(qy*qz - qx*qw);
          2*(qx*qz - qy*qw),     2*(qy*qz + qx*qw),   1 - 2*(qx^2 + qy^2) ];

    % ZYX 欧拉角
    yaw   = atan2(R(2,1), R(1,1));      % ψ (Z)
    pitch = asin(-R(3,1));              % θ (Y)
    roll  = atan2(R(3,2), R(3,3));      % φ (X)
    eul = [yaw, pitch, roll];
end

== matlab function EKF/姿态估计, 加速度映射/车体坐标, 轨道坐标估计(李群算法) ==
  data: w input; Rb output; btm_eul input; Rt output; Rtb output; R0 input
function [Rb, Rt, Rtb] = pose_update_so3(w, btm_eul, R0)
%#codegen
% Simulink版本：车体/轨道姿态估计 (SO(3))
%
% 输入:
%   w        : 3x1 体坐标角速度 [p;q;r], rad/s
%   dt       : 步长(s)，一般用采样时间常数
dt = 1e-3;
%   hasBTM   : bool, 当前步是否有 BTM 数据 (0/1)
if sum(abs(btm_eul)) > 1e-5
    hasBTM = 1;
else
    hasBTM = 0;
end
%   btm_eul  : 1x3 [yaw pitch roll], rad
%
% 输出:
%   Rb  : 3x3, 车体->世界 旋转矩阵
%   Rt  : 3x3, 轨道->世界 旋转矩阵
%   Rtb : 3x3, 轨道->车体 相对姿态矩阵

    % ===== 配置参数 (可改成 Mask 参数) =====
    beta        = 0.02;   % 轨道低通增益
    Kt          = 0.9;    % BTM 矫正增益
    onlyYaw     = false;   % 是否仅修正航向
    fixRbWithBtm= true;  % 是否同时修正 Rb
    orthoEvery  = 20;     % 每N步正交化

    % ===== persistent 状态 =====
    persistent Rb_prev Rt_prev step inited
    if isempty(inited)
        Rb_prev = R0;
        Rt_prev = R0;
        step    = 0;
        inited  = true;
    end

    % ===== 输入处理 =====
    if ~all(isfinite(w)), w(~isfinite(w)) = 0; end
    if dt < 1e-6, dt = 1e-6; end
    w = reshape(w,3,1);

    % ===== 1) 积分车体姿态 =====
    Rb_pred = Rb_prev * so3_exp(w*dt);

    % ===== 2) 轨道低通跟随 =====
    E   = Rt_prev' * Rb_pred;
    e   = so3_log(E);
    Rt_pred = Rt_prev * so3_exp(beta * e);

    % ===== 3) BTM 矫正 =====
    if hasBTM > 0.5   % true
        yaw   = btm_eul(1); pitch = btm_eul(2); roll = btm_eul(3);

        cz = cos(yaw);  sz = sin(yaw);
        cy = cos(pitch); sy = sin(pitch);
        cx = cos(roll);  sx = sin(roll);

        Rz = [cz -sz 0; sz cz 0; 0 0 1];
        Ry = [cy 0 sy; 0 1 0; -sy 0 cy];
        Rx = [1 0 0; 0 cx -sx; 0 sx cx];

        R_btm = Rz * Ry * Rx;   % body->world (若是 world->body 请改成转置)

        Et = Rt_pred' * R_btm;
        et = so3_log(Et);

        if onlyYaw
            et = [0;0;et(3)];
        end

        Rt = Rt_pred * so3_exp(Kt * et);

        if fixRbWithBtm
            Rb = Rb_pred * so3_exp(Kt * et);
        else
            Rb = Rb_pred;
        end
    else
        Rt = Rt_pred;
        Rb = Rb_pred;
    end

    % ===== 4) 数值正交化 =====
    step = step + 1;
    if mod(step, orthoEvery) == 0
        Rt = project_to_SO3(Rt);
        Rb = project_to_SO3(Rb);
    end

    % ===== 输出 =====
    Rtb    = Rt' * Rb;
    Rb_prev = Rb;
    Rt_prev = Rt;
end
















% === 辅助函数 ===
function R = so3_exp(phi)
    th = norm(phi);
    if th < 1e-12
        R = eye(3) + skew(phi);
    else
        k = phi/th;
        K = skew(k);
        R = eye(3) + sin(th)*K + (1-cos(th))*(K*K);
    end
end

function phi = so3_log(R)
    c = (trace(R)-1)/2; c = max(-1,min(1,c));
    th = acos(c);
    if th < 1e-12
        phi = [0;0;0];
        return
    end
    W = (R - R')/(2*sin(th));
    k = [W(3,2); W(1,3); W(2,1)];
    phi = th*k;
end

function S = skew(v)
    S = [  0   -v(3)  v(2);
          v(3)   0   -v(1);
         -v(2)  v(1)   0 ];
end

function R = project_to_SO3(Rin)
    [U,~,V] = svd(Rin);
    R = U*V';
    if det(R) < 0
        U(:,3) = -U(:,3);
        R = U*V';
    end
end

== matlab function EKF/姿态估计, 加速度映射/MATLAB Function2 ==
  data: Rtb input; at output; ab input
function at = fcn(Rtb, ab)
g = 9.8;
at = Rtb*ab;
at(3) = at(3)+g;
